simulink model "Closed_loop_Michelson_interferometer_v2"  (R2017b)
settings: Solver=ode3  StartTime=0.0  StopTime=0.2  FixedStep=0.00001  RelTol=1e-3  EnableMultiTasking=on
values from neighbouring files (symbols this model uses):
  A = 10    [Accelerometer_freq_response.m]    (also in Accelerometer_sensitivity_convertion.m = 5.275; Erbium_fiber_characterization_DF1500Y_15cm.m = 2.94166169712e-11; Filter_oscillating_damped_signal.m = 0.05; Laser_cavity_length_and_intensity_predictions.m = 2.46300864041e-11)
  V = 0.9507    [Accelerometer_sensitivity_convertion.m]    (also in Damping_factor_calculation.m = V_hp(sp:end))
undefined symbols (not defined in the file or in its folder): sgn
libraries: dsparch4 x1
settings Model: Creator=Roberta Martin  LastModifiedBy=Stinky
settings DataIOCC: LimitDataPoints=on  SaveFormat=Array
settings OptimizationCC: LifeSpan=inf
settings DebuggingCC: UnderspecifiedInitializationDetection=Classic  MergeDetectMultiDrivingBlocksExec=none  SolverPrmCheckMsg=warning  AllowSymbolicDim=off  SFUnexpectedBacktrackingDiag=warning  SFNoUnconditionalDefaultTransitionDiag=warning  SFExecutionAtInitializationDiag=none
settings HardwareCC: ProdBitPerPointer=32  ProdBitPerSizeT=32  ProdBitPerPtrDiffT=32  ProdLargestAtomicFloat=None  ProdIntDivRoundTo=Undefined  ProdEndianess=Unspecified  ProdWordSize=32  ProdHWDeviceType=32-bit Generic
settings ModelReferenceCC: PropagateSignalLabelsOutOfModel=off
settings CodeAppCC: StateflowObjectComments=on
settings GRTTargetCC: TargetLangStandard=C89/C90 (ANSI)  GeneratePreprocessorConditionals=Disable all
settings ConfigComp: CovMetricSettings=dw  CovHtmlReporting=on  CovSaveCumulativeToWorkspaceVar=on  CovSaveSingleToWorkspaceVar=on  CovExternalEMLEnable=off
settings SimscapeCC: SimscapeNormalizeSystem=off
settings ConfigurationSet: Description=SimMechanics 2G

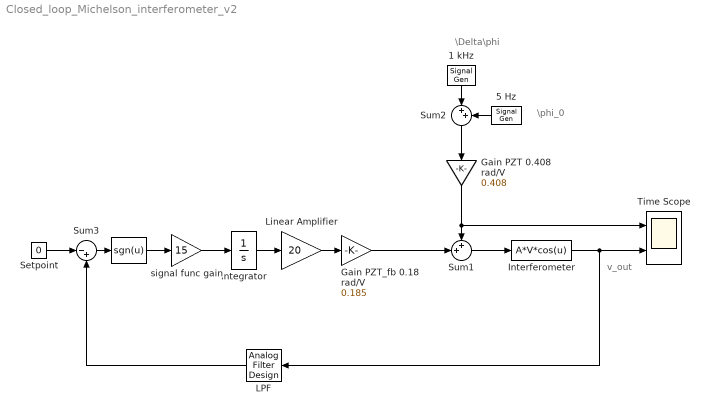
== system Closed_loop_Michelson_interferometer_v2 ==
  note: v_out
  note: \phi_0
  note: \Delta\phi
  " " : Fcn  Expr=sgn(u)
  " 5 Hz" : SignalGenerator  Amplitude=2  Frequency=5
  "1 kHz " : SignalGenerator  Frequency=1000
  Gain PZT 0.408 rad/V : Gain  Gain=0.408
  Gain PZT_fb 0.18 rad/V : Gain  Gain=0.185
  Integrator : Integrator  LimitOutput=on  UpperSaturationLimit=15  LowerSaturationLimit=-15
  Interferometer : Fcn  Expr=A*V*cos(u)
  LPF : dsparch4/Analog Filter Design  method=Butterworth  filttype=Lowpass  N=1  Wlo=20*2*pi()  Whi=80  Rp=2  Rs=40
  Linear Amplifier : Gain  Gain=20
  Setpoint : Constant  Value=0
  Sum1 : Sum  Inputs=++|
  Sum2 : Sum  Inputs=|++
  Sum3 : Sum  Inputs=|-+
  Time Scope : Scope  NumInputPorts=2
  signal func gain : Gain  Gain=15
  wires:
  Interferometer/1 -> LPF/1, Time Scope/2
  Sum1/1 -> Interferometer/1
  Linear Amplifier/1 -> Gain PZT_fb 0.18 rad/V/1
  Gain PZT 0.408 rad/V/1 -> Sum1/1, Time Scope/1
  Sum2/1 -> Gain PZT 0.408 rad/V/1
  "1 kHz "/1 -> Sum2/1
  Integrator/1 -> Linear Amplifier/1
  " 5 Hz"/1 -> Sum2/2
  Gain PZT_fb 0.18 rad/V/1 -> Sum1/2
  LPF/1 -> Sum3/2
  Sum3/1 -> " "/1
  Setpoint/1 -> Sum3/1
  " "/1 -> signal func gain/1
  signal func gain/1 -> Integrator/1
